simulink model "xianxing"  (R2022b)
settings: Solver=VariableStepAuto  StartTime=0.0  StopTime=50  RelTol=1e-3
settings Model: Creator=HONOR  LastModifiedBy=acer
settings DebuggingCC: UnconnectedInputMsg=warning  UnconnectedOutputMsg=warning  UnconnectedLineMsg=warning
settings ModelReferenceCC: EnableRefExpFcnMdlSchedulingChecks=on
settings RTWCC: DLArmComputeVersion=19.05

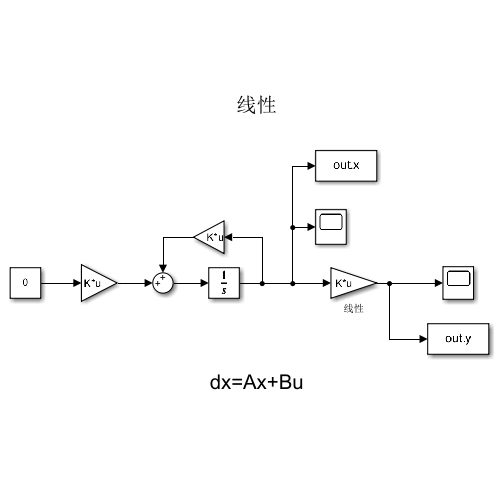
[thumbnail: Simulink's stored preview of the top-level diagram]
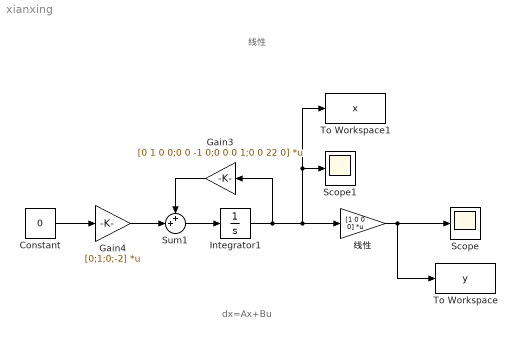
== system xianxing ==
  note: 线性
  note: dx=Ax+Bu
  Constant : Constant  Value=0
  Gain3 : Gain  Gain=[0 1 0 0;0 0 -1 0;0 0 0 1;0 0 22 0]  Multiplication=Matrix(K*u)
  Gain4 : Gain  Gain=[0;1;0;-2]  Multiplication=Matrix(K*u)
  Integrator1 : Integrator  InitialCondition=[0,0,0.1,0]
  Scope : Scope
  Scope1 : Scope
  Sum1 : Sum  Inputs=++|
  To Workspace : ToWorkspace  VariableName=y  SaveFormat=Structure With Time  SampleTime=-1
  To Workspace1 : ToWorkspace  VariableName=x  SaveFormat=Structure With Time  SampleTime=-1
  线性 : Gain  Gain=[1 0 0 0]  Multiplication=Matrix(K*u)
  wires:
  Integrator1/1 -> Gain3/1, 线性/1, To Workspace1/1, Scope1/1
  Sum1/1 -> Integrator1/1
  Gain4/1 -> Sum1/2
  线性/1 -> Scope/1, To Workspace/1
  Constant/1 -> Gain4/1
  Gain3/1 -> Sum1/1
